simulink model "Control4_SF_Vels_tiempo"  (R2023b)
settings: Solver=FixedStepAuto  StartTime=0.0  StopTime=40  RelTol=1e-3  EnableMultiTasking=on
model workspace (MAT data in the model file):
  d = 0.15
settings Model: ExtModeTrigDuration=2  Creator=Usuario  LastModifiedBy=Usuario
settings OptimizationCC: EnhancedBackFolding=on  PassReuseOutputArgsAs=Individual arguments  ZeroExternalMemoryAtStartup=off  ZeroInternalMemoryAtStartup=off  MaxStackSize=64  OptimizeBlockOrder=speed  DifferentSizesBufferReuse=on  OptimizationCustomize=off  EfficientTunableParamExpr=on
settings DebuggingCC: ParameterTunabilityLossMsg=error
settings HardwareCC: ProdBitPerInt=16  ProdBitPerPointer=16  ProdBitPerSizeT=16  ProdBitPerPtrDiffT=16  ProdLargestAtomicFloat=None  ProdWordSize=8  ProdHWDeviceType=Atmel->AVR  UseEmbeddedCoderFeatures=off  UseSimulinkCoderFeatures=off
settings SFSimCC: MATLABDynamicMemAlloc=off
settings RTWCC: Description=Embedded Coder  SystemTargetFile=ert.tlc  HardwareBoard=Arduino Mega 2560  TemplateMakefile=ert_default_tmf  Toolchain=Arduino AVR  BuildConfiguration=Faster Runs
settings CodeAppCC: ForceParamTrailComments=on  IgnoreCustomStorageClasses=off  OperatorAnnotations=on  SimulinkDataObjDesc=on  SFDataObjDesc=on  InsertBlockDesc=on
settings ERTTargetCC: SupportContinuousTime=on  SupportNonInlinedSFcns=on  SupportVariableSizeSignals=on  ExtModeTransport=3  ExtModeStaticAlloc=on  ExtModeAutomaticAllocSize=off  ExtModeStaticAllocSize=2048  ExtModeMexFile=ext_xcp  ExtModeIntrfLevel=Level2 - Open

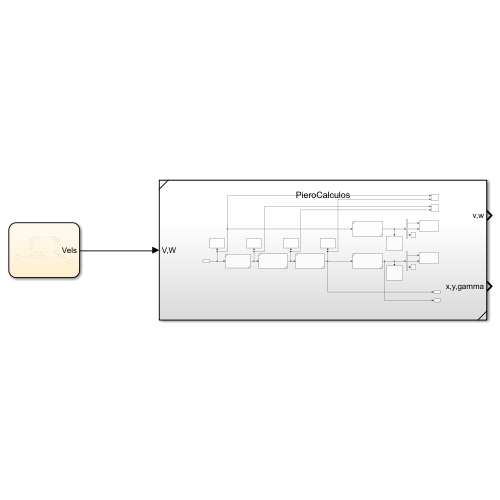
[thumbnail: Simulink's stored preview of the top-level diagram]
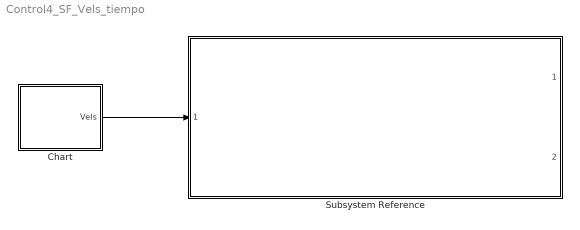
== system Control4_SF_Vels_tiempo ==
  Chart : Stateflow chart  TreatAsAtomicUnit=on
  Subsystem Reference : Subsystem  ReferencedSubsystem=PieroCalculos
  wires:
  Chart/1(Vels) -> Subsystem Reference/1

== stateflow chart Control4_SF_Vels_tiempo/Chart ==
  state Avanza3
    entry:
    Vels(1)=0.25;
    Vels(2)=0;
  state Giro2
    entry:
    Vels(1)=0;
    Vels(2)=-pi/2;
  state Giro1
    entry:
    Vels(1)=0;
    Vels(2)=-pi/2;
  state Avanza4
    entry:
    Vels(1)=0.25;
    Vels(2)=0;
  state Avanza2
    entry:
    Vels(1)=0.25;
    Vels(2)=0;
  state Giro3
    entry:
    Vels(1)=0;
    Vels(2)=pi/2;
  state Circunferencia
    entry:
    Vels(1)=0.25;
    Vels(2)=-pi/10;
  state Avanza5
    entry:
    Vels(1)=0.25;
    Vels(2)=0;
  state Inicio
    entry:
    Vels(1)=0;
    Vels(2)=0;
  state Avanza1
    entry:
    Vels(1)=0.25;
    Vels(2)=0;
  state Giro_180
    entry:
    Vels(1)=0;
    Vels(2)=-pi/2;
  state Parada
    entry:
    Vels(1)=0;
    Vels(2)=0;
  Giro2 -> Avanza4 : [after(1,sec)]
  Giro1 -> Avanza3 : [after(1,sec)]
  Avanza3 -> Giro2 : [after(6.2,sec)]
  Avanza2 -> Giro1 : [after(3.2,sec)]
  Avanza4 -> Giro3 : [after(7,sec)]
  Circunferencia -> Avanza2 : [after(5,sec)]
  Giro_180 -> Circunferencia : [after(2,sec)]
  (default) -> Inicio
  Giro3 -> Avanza5 : [after(0.5,sec)]
  Inicio -> Avanza1 : [after(1,sec)]
  Avanza5 -> Parada : [after(4,sec)]
  Avanza1 -> Giro_180 : [after(4.6,sec)]
  data: Vels output double size=2
